simulink model "lab4"  (R2024b)
settings: Solver=ode45  StartTime=0.0  StopTime=50  MaxStep=2^-5  RelTol=1e-3
libraries: simulink x2
settings Model: Creator=gm54508  LastModifiedBy=gm54508

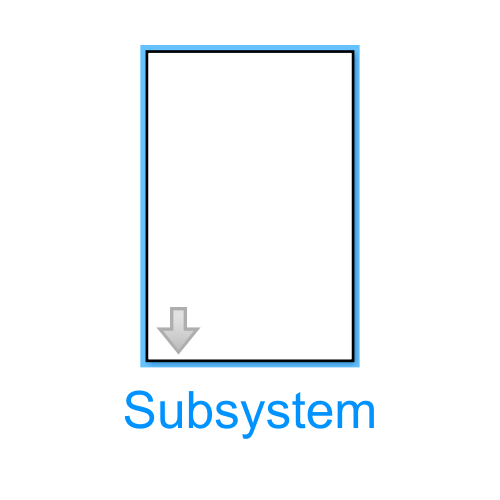
[thumbnail: Simulink's stored preview of the top-level diagram]
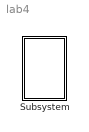
== system lab4 ==
  Subsystem : Subsystem  mask{g=9.81, m1=2.2, m2=2, M=3, R=0.002, r0=2, fi=45}

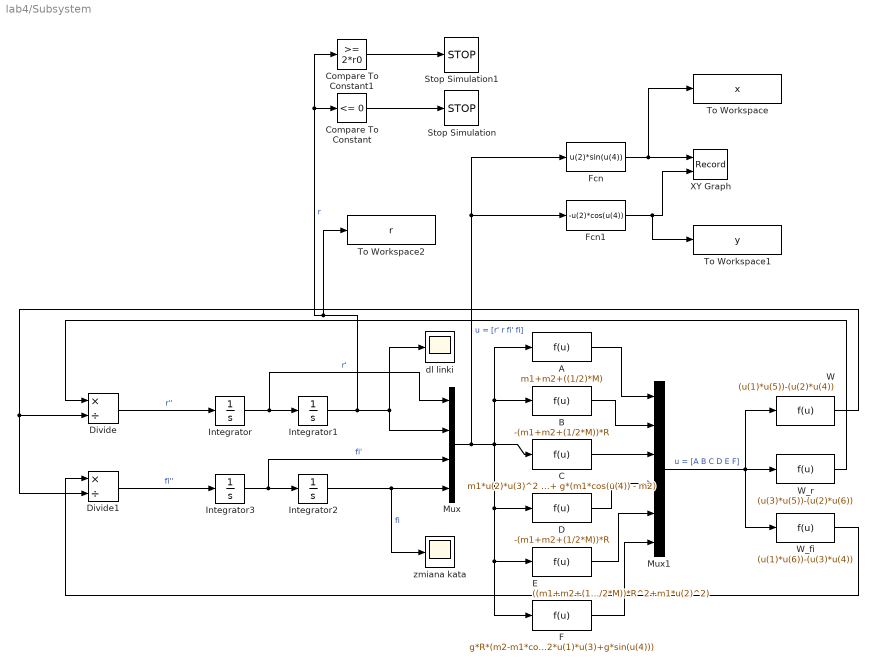
== system lab4/Subsystem ==
  A : Fcn  Expr=m1+m2+((1/2)*M)
  B : Fcn  Expr=-(m1+m2+(1/2*M))*R
  C : Fcn  Expr=m1*u(2)*u(3)^2 + g*(m1*cos(u(4)) - m2)
  Compare To Constant : simulink/Logic and Bit Operations/Compare To Constant  relop=<=  const=0  OutDataTypeStr=boolean
  Compare To Constant1 : simulink/Logic and Bit Operations/Compare To Constant  relop=>=  const=2*r0  OutDataTypeStr=boolean
  D : Fcn  Expr=-(m1+m2+(1/2*M))*R
  Divide : Product  Inputs=*/
  Divide1 : Product  Inputs=*/
  E : Fcn  Expr=((m1+m2+(1/2*M))*R^2+m1*u(2)^2)
  F : Fcn  Expr=g*R*(m2-m1*cos(u(4))) - m1*u(2)*(2*u(1)*u(3)+g*sin(u(4)))
  Fcn : Fcn  Expr=u(2)*sin(u(4))
  Fcn1 : Fcn  Expr=-u(2)*cos(u(4))
  Integrator : Integrator
  Integrator1 : Integrator  InitialCondition=r0
  Integrator2 : Integrator  InitialCondition=fi*pi/180
  Integrator3 : Integrator
  Mux : Mux
  Mux1 : Mux  Inputs=6
  Stop Simulation : Stop
  Stop Simulation1 : Stop
  To Workspace : ToWorkspace  VariableName=x  SampleTime=-1
  To Workspace1 : ToWorkspace  VariableName=y  SampleTime=-1
  To Workspace2 : ToWorkspace  VariableName=r  SampleTime=-1
  W : Fcn  Expr=(u(1)*u(5))-(u(2)*u(4))
  W_fi : Fcn  Expr=(u(1)*u(6))-(u(3)*u(4))
  W_r : Fcn  Expr=(u(3)*u(5))-(u(2)*u(6))
  XY Graph : Record  FileSettingsInternal="{\"entries\":[{\"content\":{\"excelSettings\":{\"content\":{},\"type\":\"Streamout.ExcelSettings\"}},\"type\":\"Streamout.FileSettingStorage\",\"uuid\":\"\"}],\"packageUris\":[\"http:\\/\\/schema.mathworks.com\\/mf0\\/streamout_blocks\\/R2020a\"],\"version\":\"1.0\"}"  Layout=[1 1]  SignalsInternal="{\"entries\":[{\"content\":{\"signals\":[{\"content\":{\"blockPath\":[],\"dimensions\":[1],\"domain\":\"\",\"lineColor\":\"#a2142f\",\"plots\":[ 1 ],\"port\":1,\"sid\":[\"\"],\"signalID\":1,\"signalName\":\"Fcn\"},\"type\":\"RecordBlkView.Signal\",\"uuid\":\"\"},{\"content\":{\"blockPath\":[],\"dimensions\":[1],\"domain\":\"\",\"lineColor\":\"#139fff\",\"plots\":[ 1 ],\"port\":2,\"sid\":[\"\"],\"signalID\":2,\"signalName\":\"Fcn1\"},\"type\":\"RecordBlkView.Signal\",\"uuid\":\"\"}]},\"type\":\"RecordBlkView.InputSignals\",\"uuid\":\"\"}],\"packageUris\":[\"http:\\/\\/schema.mathworks.com\\/mf0\\/streamout_blocks\\/R2020a\"],\"version\":\"1.0\"}"  VisualizationBindings="{\"xyplotplugin\":{\"info\":[{\"series\":[{\"bindingParametersList\":[{\"parameter\":\"X-Axis\",\"signalID\":1,\"signalName\":\"Fcn\"},{\"parameter\":\"Y-Axis\",\"signalID\":2,\"signalName\":\"Fcn1\"}],\"seriesID\":0}],\"subplotID\":1}]}}"  CompatibilityTag=XY
  dl linki : Scope
  zmiana kata : Scope
  wires:
  Integrator/1 -> Mux/1, Integrator1/1  "r'"
  E/1 -> Mux1/5
  Mux1/1 -> W_fi/1, W_r/1, W/1  "u = [A B C D E F]"
  Integrator3/1 -> Mux/3, Integrator2/1  "fi'"
  Mux/1 -> Fcn1/1, Fcn/1, C/1, F/1, E/1, D/1, B/1, A/1  "u = [r' r fi' fi]"
  C/1 -> Mux1/3
  B/1 -> Mux1/2
  D/1 -> Mux1/4
  W/1 -> Divide1/2, Divide/2
  Integrator1/1 -> To Workspace2/1, Compare To Constant1/1, Compare To Constant/1, Mux/2, dl linki/1  "r"
  A/1 -> Mux1/1
  Integrator2/1 -> zmiana kata/1, Mux/4  "fi"
  W_fi/1 -> Divide1/1
  Divide1/1 -> Integrator3/1  "fi''"
  W_r/1 -> Divide/1
  Divide/1 -> Integrator/1  "r''"
  F/1 -> Mux1/6
  Fcn1/1 -> To Workspace1/1, XY Graph/2
  Fcn/1 -> To Workspace/1, XY Graph/1
  Compare To Constant/1 -> Stop Simulation/1
  Compare To Constant1/1 -> Stop Simulation1/1
